simulink model "car_model"  (R2017a)
settings: Solver=ode8  StartTime=0.0  StopTime=tf  FixedStep=1e-3  RelTol=1e-3  AbsTol=1e-6
values from neighbouring files (symbols this model uses):
  sys = kinematic_model(sys)    [load_kin.m]
undefined symbols (not defined in the file or in its folder): L, MAX_DELTA, w, x0
(part 1 of 2)
settings Model: Creator=brunolnetto  LastModifiedBy=brunolnetto
settings DataIOCC: SaveState=on  StateSaveName=xoutNew  OutputSaveName=youtNew

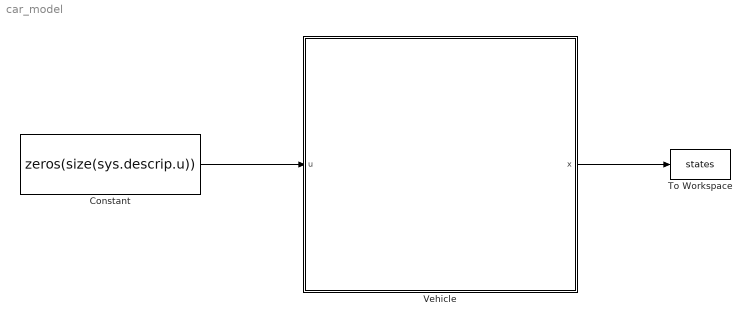
== system car_model ==
  Constant : Constant  Value=zeros(size(sys.descrip.u))
  To Workspace : ToWorkspace  VariableName=states  SaveFormat=Structure With Time  SampleTime=-1
  Vehicle : Subsystem
      mask Display: image('/home/brunolnetto/Pictures/auto_model.png');
  wires:
  Constant/1 -> Vehicle/1(u)
  Vehicle/1(x) -> To Workspace/1

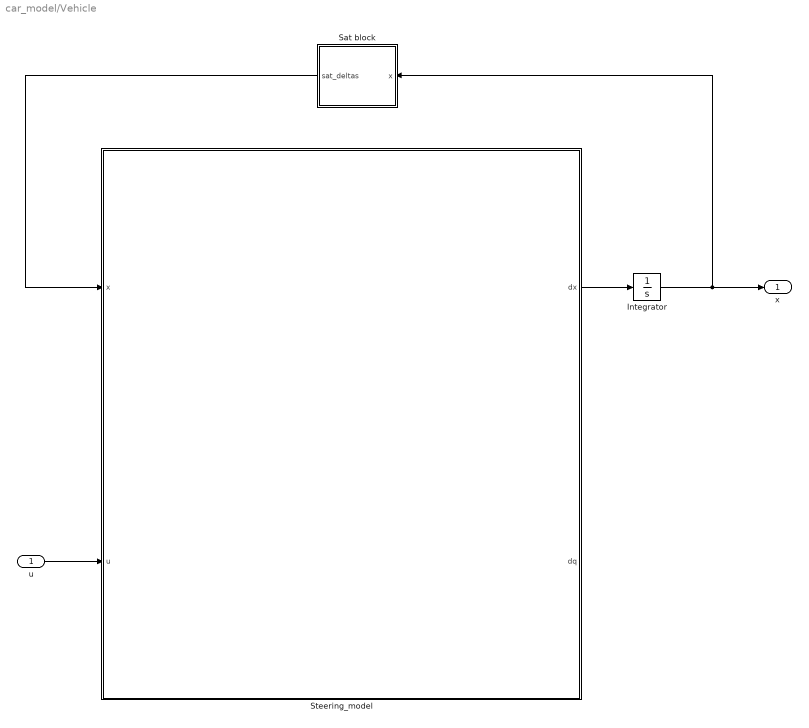
== system car_model/Vehicle ==
  u : Inport
  Integrator : Integrator  InitialCondition=x0
  Sat block : Subsystem
  Steering_model : Subsystem
      mask Display: image('/home/brunolnetto/Pictures/steer_schema.png');
  x : Outport
  wires:
  Steering_model/1(dx) -> Integrator/1
  u/1 -> Steering_model/2(u)
  Integrator/1 -> Sat block/1(x), x/1
  Sat block/1(sat_deltas) -> Steering_model/1(x)

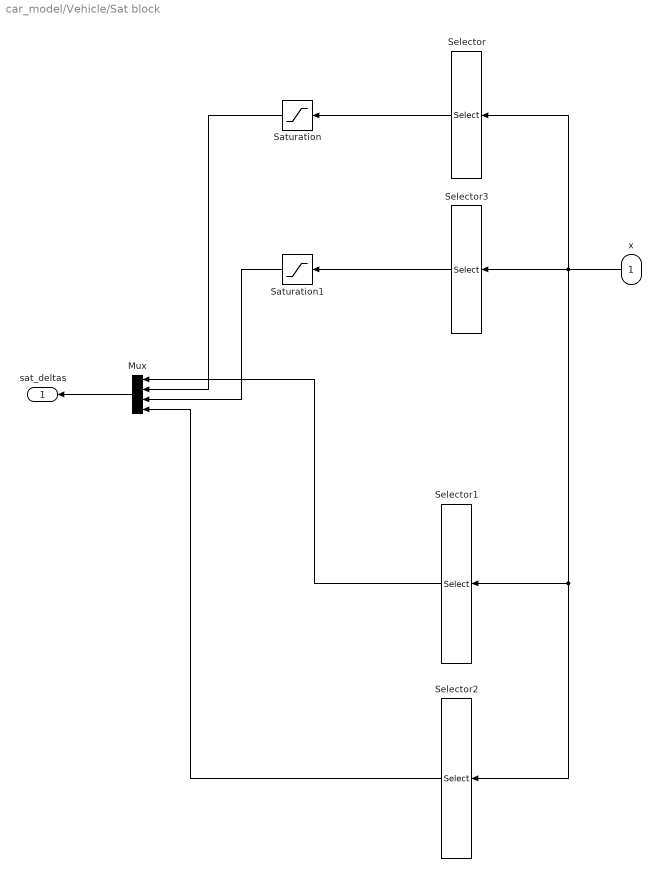
== system car_model/Vehicle/Sat block ==
  x : Inport
  Mux : Mux
  Saturation : Saturate  UpperLimit=MAX_DELTA  LowerLimit=atan(tan(-MAX_DELTA)/(1 - (w/L)*tan(-MAX_DELTA)))
  Saturation1 : Saturate  UpperLimit=atan(tan(MAX_DELTA)/(1 + (w/L)*tan(MAX_DELTA)))  LowerLimit=-MAX_DELTA
  Selector : Selector  InputPortWidth=13  IndexOptions=Index vector (dialog)  Indices=4  OutputSizes=1
  Selector1 : Selector  InputPortWidth=13  IndexOptions=Index vector (dialog)  Indices=[1 2. 3]  OutputSizes=1
  Selector2 : Selector  InputPortWidth=13  IndexOptions=Index vector (dialog)  Indices=[6. 7. 8. 9. 10. 11. 12. 13]  OutputSizes=1
  Selector3 : Selector  InputPortWidth=13  IndexOptions=Index vector (dialog)  Indices=5  OutputSizes=1
  sat_deltas : Outport
  wires:
  Selector/1 -> Saturation/1
  Mux/1 -> sat_deltas/1
  x/1 -> Selector2/1, Selector1/1, Selector3/1, Selector/1
  Selector3/1 -> Saturation1/1
  Selector2/1 -> Mux/4
  Selector1/1 -> Mux/1
  Saturation/1 -> Mux/2
  Saturation1/1 -> Mux/3

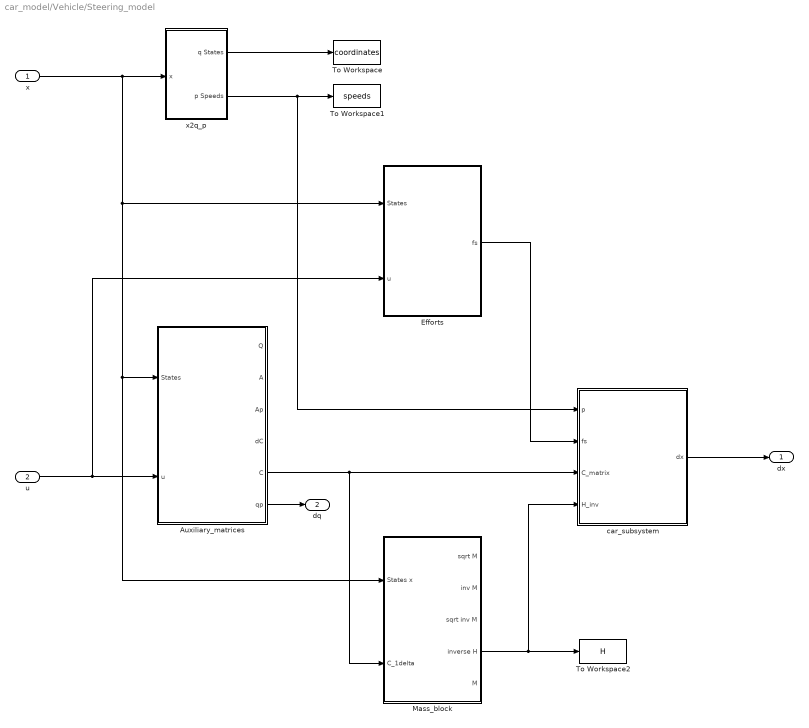
== system car_model/Vehicle/Steering_model ==
  x : Inport
  u : Inport  Port=2
  Auxiliary_matrices : Subsystem
  Efforts : Subsystem
  Mass_block : Subsystem
  To Workspace : ToWorkspace  VariableName=coordinates  SaveFormat=Structure With Time  SampleTime=-1
  To Workspace1 : ToWorkspace  VariableName=speeds  SaveFormat=Structure With Time  SampleTime=-1
  To Workspace2 : ToWorkspace  VariableName=H  SaveFormat=Structure With Time  SampleTime=-1
  car_subsystem : Subsystem
  x2q_p : Subsystem
  dx : Outport
  dq : Outport  Port=2
  wires:
  Auxiliary_matrices/5(C) -> Mass_block/2("C_1delta  "), car_subsystem/3(C_matrix)
  u/1 -> Efforts/2(u), Auxiliary_matrices/2(u)
  Mass_block/4(inverse H) -> To Workspace2/1, car_subsystem/4(H_inv)
  car_subsystem/1(dx) -> dx/1
  Efforts/1(fs) -> car_subsystem/2(fs)
  x2q_p/1(q States) -> To Workspace/1
  x2q_p/2(p Speeds) -> To Workspace1/1, car_subsystem/1(p)
  x/1 -> x2q_p/1(x), Mass_block/1(States x), Auxiliary_matrices/1(States), Efforts/1(States)
  Auxiliary_matrices/6(qp) -> dq/1

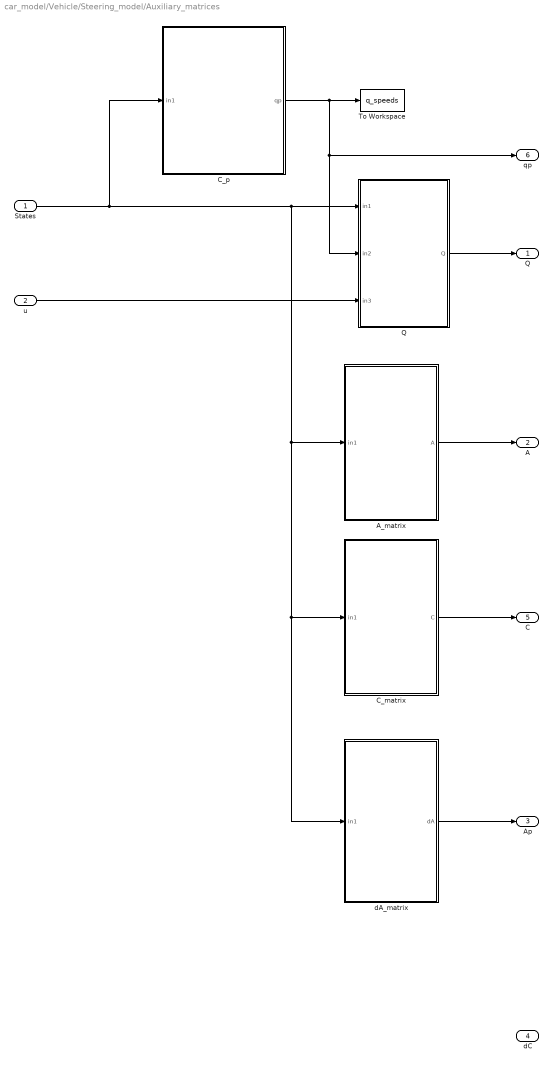
== system car_model/Vehicle/Steering_model/Auxiliary_matrices ==
  States : Inport
  u : Inport  Port=2
  A_matrix : MATLAB Function  TreatAsAtomicUnit=on
  C_matrix : MATLAB Function  TreatAsAtomicUnit=on
  C_p : MATLAB Function  TreatAsAtomicUnit=on
  Q : MATLAB Function  TreatAsAtomicUnit=on
  To Workspace : ToWorkspace  VariableName=q_speeds  SaveFormat=Structure With Time  SampleTime=-1
  dA_matrix : MATLAB Function  TreatAsAtomicUnit=on
  "Q " : Outport
  A : Outport  Port=2
  Ap : Outport  Port=3
  dC : Outport  Port=4
  C : Outport  Port=5
  qp : Outport  Port=6
  wires:
  C_matrix/1(C) -> C/1
  Q/1(Q) -> "Q "/1
  A_matrix/1(A) -> A/1
  dA_matrix/1(dA) -> Ap/1
  u/1 -> Q/3(in3)
  States/1 -> C_p/1(in1), dA_matrix/1(in1), C_matrix/1(in1), A_matrix/1(in1), Q/1(in1)
  C_p/1(qp) -> To Workspace/1, qp/1, Q/2(in2)

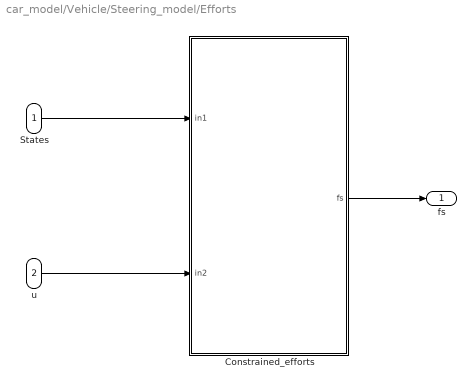
== system car_model/Vehicle/Steering_model/Efforts ==
  States : Inport
  u : Inport  Port=2
  Constrained_efforts : MATLAB Function  TreatAsAtomicUnit=on
  fs : Outport
  wires:
  States/1 -> Constrained_efforts/1(in1)
  u/1 -> Constrained_efforts/2(in2)
  Constrained_efforts/1(fs) -> fs/1

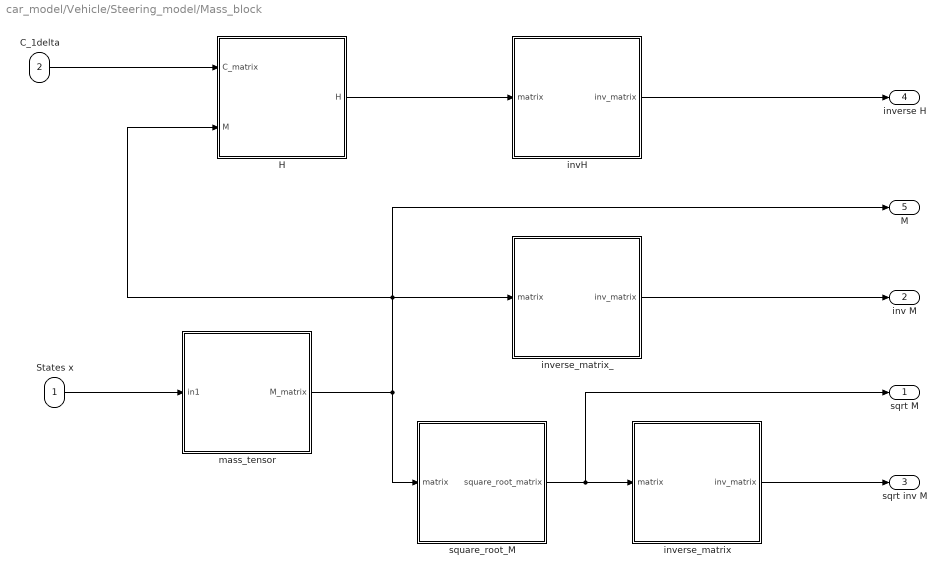
== system car_model/Vehicle/Steering_model/Mass_block ==
  States x : Inport
  "C_1delta  " : Inport  Port=2
  H : MATLAB Function  TreatAsAtomicUnit=on
  invH : MATLAB Function  TreatAsAtomicUnit=on
  inverse_matrix : MATLAB Function  TreatAsAtomicUnit=on
  inverse_matrix_ : MATLAB Function  TreatAsAtomicUnit=on
  mass_tensor : MATLAB Function  TreatAsAtomicUnit=on
  square_root_M : MATLAB Function  TreatAsAtomicUnit=on
  sqrt M : Outport
  inv M : Outport  Port=2
  sqrt inv M : Outport  Port=3
  inverse H : Outport  Port=4
  M : Outport  Port=5
  wires:
  States x/1 -> mass_tensor/1(in1)
  "C_1delta  "/1 -> H/1(C_matrix)
  inverse_matrix_/1(inv_matrix) -> inv M/1
  H/1(H) -> invH/1(matrix)
  invH/1(inv_matrix) -> inverse H/1
  inverse_matrix/1(inv_matrix) -> sqrt inv M/1
  mass_tensor/1(M_matrix) -> M/1, inverse_matrix_/1(matrix), H/2(M), square_root_M/1(matrix)
  square_root_M/1(square_root_matrix) -> sqrt M/1, inverse_matrix/1(matrix)

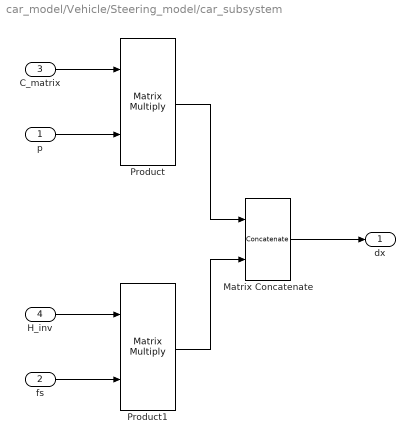
== system car_model/Vehicle/Steering_model/car_subsystem ==
  p : Inport
  fs : Inport  Port=2
  C_matrix : Inport  Port=3
  H_inv : Inport  Port=4
  Matrix Concatenate : Concatenate  ConcatenateDimension=2
  Product : Product  Multiplication=Matrix(*)
  Product1 : Product  Multiplication=Matrix(*)
  dx : Outport
  wires:
  Product/1 -> Matrix Concatenate/1
  p/1 -> Product/2
  C_matrix/1 -> Product/1
  Product1/1 -> Matrix Concatenate/2
  H_inv/1 -> Product1/1
  fs/1 -> Product1/2
  Matrix Concatenate/1 -> dx/1

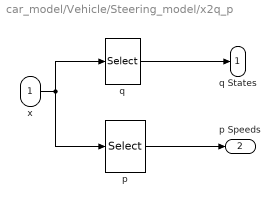
== system car_model/Vehicle/Steering_model/x2q_p ==
  x : Inport
  p : Selector  InputPortWidth=13  IndexOptions=Index vector (dialog)  Indices=[10 11 12 13]  OutputSizes=1
  q : Selector  InputPortWidth=13  IndexOptions=Index vector (dialog)  Indices=[1 2 3 4 5 6 7 8 9]  OutputSizes=1
  q States : Outport
  p Speeds : Outport  Port=2
  wires:
  x/1 -> p/1, q/1
  q/1 -> q States/1
  p/1 -> p Speeds/1

== matlab function car_model/Vehicle/Steering_model/Auxiliary_matrices/A_matrix ==
  data: in1 input; A output
function A = ConstraintMatrix(in1)

%    This function was generated by the Symbolic Math Toolbox version 7.2.

%    11-Nov-2020 11:00:00



delta_o = in1(5,:);

theta = in1(3,:);

t2 = tan(theta);

t3 = tan(delta_o);

t4 = t2.*(3.0./2.0);

t5 = t4+9.0./2.0;

t6 = 1.0./t5;

t7 = t2.^2;

t8 = 1.0./t5.^2;

t9 = t7.*t8.*(8.1e1./4.0);

t10 = t9+1.0;

t11 = t2.*t6.*(2.7e1./4.0);

t12 = t2.*t6.*(9.0./2.0);

t13 = atan(t12);

t14 = t13+theta;

t15 = 1.0./sqrt(t10);

t16 = sin(t14);

t17 = cos(t14);

A = reshape([0.0,0.0,0.0,t17,-t16,0.0,0.0,0.0,t16,t17,0.0,0.0,0.0,t15.*(-9.0./2.0)+t2.*t6.*t15.*(2.7e1./8.0),t15.*(3.0./4.0)+t2.*t6.*t15.*(8.1e1./4.0),t10.*(t3.*(3.0./2.0)-9.0./2.0).*(-2.0./9.0),0.0,0.0,0.0,0.0,(t3.^2+1.0).*(t11+9.0./2.0).*(-2.0./9.0),0.0,0.0,0.0,0.0,0.0,0.0,sqrt(t10),-3.442462000000001e-1,0.0,0.0,0.0,(t11-9.0)./(cos(delta_o).*(t11+9.0)),0.0,0.0,0.0,t2.*t6.*(-3.0./2.0)-1.0,0.0,0.0,0.0,0.0,1.0,0.0,0.0,0.0],[5,9]);

end

== matlab function car_model/Vehicle/Steering_model/Mass_block/mass_tensor ==
  data: in1 input; M_matrix output
function M_matrix = Mass_matrix(in1)

%    This function was generated by the Symbolic Math Toolbox version 7.2.

%    11-Nov-2020 11:00:06



delta_o = in1(5,:);

phi_i = in1(6,:);

phi_l = in1(9,:);

phi_o = in1(7,:);

phi_r = in1(8,:);

theta = in1(3,:);

t2 = cos(theta);

t3 = sin(theta);

t4 = cos(phi_i);

t5 = t4.^2;

t6 = cos(phi_l);

t7 = t6.^2;

t8 = cos(phi_o);

t9 = t8.^2;

t10 = cos(phi_r);

t11 = t10.^2;

t12 = t2.^2;

t13 = sin(phi_l);

t14 = t13.^2;

t15 = sin(phi_r);

t16 = t15.^2;

t17 = t3.^2;

t18 = cos(delta_o);

t19 = sin(phi_o);

t20 = t19.^2;

t21 = t18.^2;

t22 = sin(delta_o);

t23 = t22.^2;

t24 = t20.^2;

t25 = sin(phi_i);

t26 = t25.^2;

t27 = tan(theta);

t28 = t27.^2;

t29 = t27.*(3.0./2.0);

t30 = t29+9.0./2.0;

t31 = 1.0./t30.^2;

t32 = t28.*t31.*(8.1e1./4.0);

t33 = t32+1.0;

t34 = 1.0./t33;

t35 = t26.^2;

t36 = 1.0./sqrt(t33);

t37 = 1.0./t30;

t38 = phi_i.*4.0;

t39 = cos(t38);

t40 = t5.^2;

t41 = t40.*4.147690617505401e-1;

t42 = t12.*t34.*t35.*4.147690617505401e-1;

t43 = t17.*t26.*t34.*2.073845308752701e-1;

t44 = t5.*t12.*t26.*t34.*2.073845308752701e-1;

t45 = t12.*t26.*t28.*t31.*t34.*4.199536750224219;

t46 = t17.*t28.*t31.*t34.*t35.*8.399073500448438;

t47 = t3.*t5.*t26.*t27.*t36.*t37.*1.866460777877431;

t48 = t2.*t3.*t26.*t27.*t34.*t37.*1.866460777877431;

t49 = t5.*t17.*t26.*t28.*t31.*t34.*4.199536750224219;

t50 = phi_o.*4.0;

t51 = cos(t50);

t52 = t9.^2;

t53 = t52.*4.147690617505401e-1;

t54 = t12.*t21.*t24.*4.147690617505401e-1;

t55 = t17.*t20.*t21.*2.073845308752701e-1;

t56 = t12.*t20.*t23.*2.073845308752701e-1;

t57 = t17.*t23.*t24.*4.147690617505401e-1;

t58 = t9.*t12.*t20.*t21.*2.073845308752701e-1;

t59 = t9.*t17.*t20.*t23.*2.073845308752701e-1;

t60 = t3.*t9.*t20.*t22.*4.147690617505401e-1;

t61 = t2.*t3.*t18.*t20.*t22.*4.147690617505401e-1;

t62 = phi_i.*3.0;

t63 = sin(t62);

t64 = theta.*2.0;

t65 = t27.*t37.*(9.0./2.0);

t66 = atan(t65);

t67 = t66.*2.0;

t68 = cos(t64);

t69 = sin(t67);

t70 = sin(t64);

t71 = cos(t67);

t72 = delta_o.*2.0;

t73 = phi_o.*3.0;

t74 = sin(t73);

t75 = cos(t72);

t76 = sin(t72);

t78 = t39.*2.592306635940876e-2;

t79 = t2.*t5.*t26.*t36.*4.147690617505401e-1;

t80 = t2.*t3.*t27.*t34.*t35.*t37.*3.732921555754861;

t81 = t2.*t3.*t5.*t26.*t27.*t34.*t37.*1.866460777877431;

t77 = t41+t42+t43+t44+t45+t46+t47+t48+t49-t78-t79-t80-t81+2.592306635940876e-2;

t82 = t63.*t68.*t69.*2.592306635940876e-2;

t83 = t63.*t70.*t71.*2.592306635940876e-2;

t84 = t3.*t25.*t36.*5.184613271881752e-2;

t85 = t3.*t36.*t63.*5.184613271881752e-2;

t86 = t2.*t25.*t27.*t36.*t37.*2.333075972346788e-1;

t87 = t2.*t27.*t36.*t37.*t63.*2.333075972346788e-1;

t101 = t25.*t68.*t69.*7.776919907822627e-2;

t102 = t25.*t70.*t71.*7.776919907822627e-2;

t88 = t82+t83+t84+t85+t86+t87-t101-t102;

t90 = t51.*2.592306635940876e-2;

t91 = t2.*t9.*t18.*t20.*4.147690617505401e-1;

t92 = t2.*t3.*t18.*t22.*t24.*8.295381235010802e-1;

t93 = t2.*t3.*t9.*t18.*t20.*t22.*4.147690617505401e-1;

t89 = t53+t54+t55+t56+t57+t58+t59+t60+t61-t90-t91-t92-t93+2.592306635940876e-2;

t94 = t70.*t74.*t75.*2.592306635940876e-2;

t95 = t68.*t74.*t76.*2.592306635940876e-2;

t96 = t3.*t18.*t74.*5.184613271881752e-2;

t97 = t2.*t22.*t74.*5.184613271881752e-2;

t98 = t3.*t18.*t19.*5.184613271881752e-2;

t99 = t2.*t19.*t22.*5.184613271881752e-2;

t103 = t19.*t70.*t75.*7.776919907822627e-2;

t104 = t19.*t68.*t76.*7.776919907822627e-2;

t100 = t94+t95+t96+t97+t98+t99-t103-t104;

t105 = t2.*t3.*t15.*2.073845308752701e-1;

t106 = t3.*t11.*t15.*2.073845308752701e-1;

t107 = t105+t106-t2.*t3.*t11.*t15.*2.073845308752701e-1-t2.*t3.*t15.*t16.*4.147690617505401e-1;

t108 = t2.*t3.*t13.*2.073845308752701e-1;

t109 = t3.*t7.*t13.*2.073845308752701e-1;

t110 = t108+t109-t2.*t3.*t7.*t13.*2.073845308752701e-1-t2.*t3.*t13.*t14.*4.147690617505401e-1;

t111 = t12.*2.073845308752701e-1;

M_matrix = reshape([1.885e3,0.0,t2.*(-4.24125e3),0.0,0.0,0.0,0.0,0.0,0.0,0.0,1.885e3,t3.*(-4.24125e3),0.0,0.0,0.0,0.0,0.0,0.0,t2.*(-4.24125e3),t3.*(-4.24125e3),t12.*9.7003125e3+t17.*9.7003125e3-t39.*2.592306635940876e-2+t41+t42+t43+t44+t45+t46+t47+t48+t49-t51.*2.592306635940876e-2+t53+t54+t55+t56+t57+t58+t59+t60+t61-cos(phi_l.*4.0).*2.592306635940876e-2-cos(phi_r.*4.0).*2.592306635940876e-2+t14.*t17.*2.073845308752701e-1+t16.*t17.*2.073845308752701e-1+t12.*t14.^2.*4.147690617505401e-1+t12.*t16.^2.*4.147690617505401e-1+t7.^2.*4.147690617505401e-1+t11.^2.*4.147690617505401e-1+t2.*t7.*(t7-1.0).*4.147690617505401e-1+t2.*t11.*(t11-1.0).*4.147690617505401e-1+t7.*t12.*t14.*2.073845308752701e-1+t11.*t12.*t16.*2.073845308752701e-1-t2.*t9.*t18.*t20.*4.147690617505401e-1-t2.*t5.*t26.*t36.*4.147690617505401e-1-t2.*t3.*t18.*t22.*t24.*8.295381235010802e-1-t2.*t3.*t9.*t18.*t20.*t22.*4.147690617505401e-1-t2.*t3.*t27.*t34.*t35.*t37.*3.732921555754861-t2.*t3.*t5.*t26.*t27.*t34.*t37.*1.866460777877431+3.481978692265438e3,t77,t89,t88,t100,t107,t110,0.0,0.0,t77,t77,0.0,t88,0.0,0.0,0.0,0.0,0.0,t89,0.0,t89,0.0,t100,0.0,0.0,0.0,0.0,t88,t88,0.0,t5.*(-1.03692265437635e-1)-t68.*t71.*1.03692265437635e-1+t69.*t70.*1.03692265437635e-1+t5.*t68.*t71.*1.03692265437635e-1-t5.*t69.*t70.*1.03692265437635e-1+3.110767963129051e-1,0.0,0.0,0.0,0.0,0.0,t100,0.0,t100,0.0,t9.*(-1.03692265437635e-1)-t68.*t75.*1.03692265437635e-1+t70.*t76.*1.03692265437635e-1+t9.*t68.*t75.*1.03692265437635e-1-t9.*t70.*t76.*1.03692265437635e-1+3.110767963129051e-1,0.0,0.0,0.0,0.0,t107,0.0,0.0,0.0,0.0,t111+t11.*t17.*2.073845308752701e-1+t16.*t17.*4.147690617505401e-1,0.0,0.0,0.0,t110,0.0,0.0,0.0,0.0,0.0,t111+t7.*t17.*2.073845308752701e-1+t14.*t17.*4.147690617505401e-1],[9,9]);

end

== matlab function car_model/Vehicle/Steering_model/Auxiliary_matrices/C_matrix ==
  data: in1 input; C output
function C = KinematicMatrix(in1)

%    This function was generated by the Symbolic Math Toolbox version 7.2.

%    11-Nov-2020 11:00:01



delta_o = in1(5,:);

theta = in1(3,:);

t2 = tan(theta);

t3 = t2.^2;

t4 = t2.*(3.0./2.0);

t5 = t4+9.0./2.0;

t6 = 1.0./t5.^2;

t7 = t3.*t6.*(8.1e1./4.0);

t8 = t7+1.0;

t9 = 1.0./sqrt(t8);

t10 = 1.0./t5;

t11 = t2.*t10.*(9.0./2.0);

t12 = atan(t11);

t13 = t12.*2.0;

t14 = t13+theta;

t15 = cos(theta);

t16 = t15.*(9.0./2.0);

t17 = sin(theta);

t18 = t17.*(3.0./4.0);

t19 = cos(delta_o);

t20 = 1.0./t19;

t21 = t9.*9.0;

t22 = t2.*t9.*t10.*(2.7e1./4.0);

t23 = t21+t22;

t24 = 1.0./t23;

t25 = cos(t14);

t26 = sin(t14);

t27 = t17.*(9.0./2.0);

t28 = delta_o.*2.0;

C = reshape([t16+t18,t15.*(-3.0./4.0)+t27,1.0,0.0,0.0,0.0,0.0,0.0,0.0,0.0,0.0,0.0,(cos(t13).*(9.0./2.0)+sin(t13).*(3.0./2.0)+9.0./2.0)./(cos(t28).*(9.0./2.0)-sin(t28).*(3.0./2.0)+9.0./2.0),1.0,0.0,0.0,0.0,0.0,t9.*t20.*t24.*(t16+t18+t25.*(9.0./2.0)-t26.*(3.0./4.0)).*3.442462000000001e-1,t9.*t20.*t24.*(t15.*(-3.0./4.0)+t25.*(3.0./4.0)+t26.*(9.0./2.0)+t27).*3.442462000000001e-1,0.0,0.0,0.0,t9.*t20.*t24.*(t21-t22),1.0,0.0,0.0,0.0,0.0,0.0,0.0,0.0,0.0,0.0,(9.0./2.0)./(t2.*t10.*(2.7e1./4.0)+9.0./2.0),1.0],[9,4]);

end

== matlab function car_model/Vehicle/Steering_model/Auxiliary_matrices/Q ==
  data: in1 input; in2 input; in3 input; Q output
function Q = EffortVector(in1,in2,in3)

%    This function was generated by the Symbolic Math Toolbox version 7.2.

%    11-Nov-2020 10:59:58



delta_o = in1(5,:);

deltap_i = in2(4,:);

deltap_o = in2(5,:);

f_phi_i = in3(1,:);

f_phi_l = in3(4,:);

f_phi_o = in3(2,:);

f_phi_r = in3(3,:);

phi_i = in1(6,:);

phi_l = in1(9,:);

phi_o = in1(7,:);

phi_r = in1(8,:);

phip_i = in2(6,:);

phip_l = in2(9,:);

phip_o = in2(7,:);

phip_r = in2(8,:);

thetap = in2(3,:);

theta = in1(3,:);

t2 = thetap.^2;

t3 = sin(theta);

t4 = tan(theta);

t5 = t4.*(3.0./2.0);

t6 = t5+9.0./2.0;

t7 = 1.0./t6;

t8 = t4.*t7.*(9.0./2.0);

t9 = atan(t8);

t10 = t9+theta;

t11 = sin(t10);

t12 = phip_l.^2;

t13 = theta.*2.0;

t14 = phip_r.^2;

t15 = phip_o.^2;

t16 = delta_o.*2.0;

t17 = deltap_o.^2;

t18 = phi_o.*2.0;

t19 = t13+t16+t18;

t20 = sin(t19);

t21 = t13+t16-t18;

t22 = sin(t21);

t23 = phi_o.*4.0;

t24 = t13+t16+t23;

t25 = sin(t24);

t26 = sin(t13);

t27 = phip_i.^2;

t28 = t13+t16;

t29 = sin(t28);

t30 = phi_l.*2.0;

t31 = phi_l.*3.0;

t32 = phi_r.*2.0;

t33 = phi_r.*3.0;

t34 = -t13+t30;

t35 = sin(t34);

t36 = t13+t30;

t37 = sin(t36);

t38 = phi_l.*4.0;

t39 = -t13+t32;

t40 = sin(t39);

t41 = t13+t32;

t42 = sin(t41);

t43 = phi_r.*4.0;

t44 = deltap_i.^2;

t45 = t9.*2.0;

t46 = phi_o.*3.0;

t47 = delta_o-t23+theta;

t48 = sin(t47);

t49 = delta_o+t23+theta;

t50 = sin(t49);

t51 = phi_i.*2.0;

t52 = t13+t45+t51;

t53 = sin(t52);

t54 = t13+t45-t51;

t55 = sin(t54);

t56 = phi_i.*4.0;

t57 = t13+t45+t56;

t58 = sin(t57);

t59 = delta_o+theta;

t60 = sin(t59);

t61 = t13+t45;

t62 = sin(t61);

t63 = phi_i.*3.0;

t64 = t9-t56+theta;

t65 = sin(t64);

t66 = t9+t56+theta;

t67 = sin(t66);

t68 = t38+theta;

t69 = sin(t68);

t70 = t43+theta;

t71 = sin(t70);

t72 = t13+t16-t23;

t73 = sin(t72);

t74 = sin(t51);

t75 = sin(t56);

t76 = sin(t18);

t77 = sin(t23);

t78 = t38-theta;

t79 = sin(t78);

t80 = -t13+t38;

t81 = sin(t80);

t82 = t13+t38;

t83 = sin(t82);

t84 = t43-theta;

t85 = sin(t84);

t86 = -t13+t43;

t87 = sin(t86);

t88 = t13+t43;

t89 = sin(t88);

t90 = t13+t45-t56;

t91 = sin(t90);

t92 = phi_i+t13+t45;

t93 = sin(t92);

t94 = t27.*t93.*3.888459953911314e-2;

t95 = phi_i+t9+theta;

t96 = sin(t95);

t97 = t44.*t58.*6.480766589852189e-3;

t98 = -phi_i+t13+t45;

t99 = sin(t98);

t100 = t27.*t99.*3.888459953911314e-2;

t101 = t13+t45+t63;

t102 = sin(t101);

t103 = t2.*t91.*6.480766589852189e-3;

t104 = t2.*t58.*6.480766589852189e-3;

t105 = t44.*t62.*3.888459953911314e-2;

t106 = t27.*t62.*5.184613271881752e-2;

t107 = t2.*t62.*3.888459953911314e-2;

t108 = t44.*t65.*1.296153317970438e-2;

t109 = t44.*t67.*1.296153317970438e-2;

t110 = -phi_i+t9+theta;

t111 = sin(t110);

t112 = t9-t63+theta;

t113 = sin(t112);

t114 = t9+t63+theta;

t115 = sin(t114);

t116 = t2.*t65.*1.296153317970438e-2;

t117 = t2.*t67.*1.296153317970438e-2;

t118 = deltap_i.*t65.*thetap.*2.592306635940876e-2;

t119 = deltap_i.*t67.*thetap.*2.592306635940876e-2;

t120 = phip_i.*t67.*thetap.*1.03692265437635e-1;

t121 = deltap_i.*phip_i.*t74.*1.03692265437635e-1;

t122 = deltap_i.*phip_i.*t75.*1.555383981564525e-1;

t123 = phip_i.*t74.*thetap.*1.03692265437635e-1;

t124 = phip_i.*t75.*thetap.*1.555383981564525e-1;

t125 = deltap_i.*phip_i.*t55.*5.184613271881752e-2;

t126 = deltap_i.*phip_i.*t58.*2.592306635940876e-2;

t127 = deltap_i.*t91.*thetap.*1.296153317970438e-2;

t128 = deltap_i.*t58.*thetap.*1.296153317970438e-2;

t129 = phip_i.*t55.*thetap.*5.184613271881752e-2;

t130 = phip_i.*t58.*thetap.*2.592306635940876e-2;

t131 = deltap_i.*t62.*thetap.*7.776919907822627e-2;

t132 = deltap_i.*phip_i.*t67.*1.03692265437635e-1;

t133 = phi_o+t13+t16;

t134 = sin(t133);

t135 = t15.*t134.*3.888459953911314e-2;

t136 = delta_o+phi_o+theta;

t137 = sin(t136);

t138 = t17.*t25.*6.480766589852189e-3;

t139 = -phi_o+t13+t16;

t140 = sin(t139);

t141 = t15.*t140.*3.888459953911314e-2;

t142 = t13+t16+t46;

t143 = sin(t142);

t144 = t2.*t73.*6.480766589852189e-3;

t145 = t2.*t25.*6.480766589852189e-3;

t146 = t17.*t29.*3.888459953911314e-2;

t147 = t15.*t29.*5.184613271881752e-2;

t148 = t2.*t29.*3.888459953911314e-2;

t149 = t17.*t48.*1.296153317970438e-2;

t150 = t17.*t50.*1.296153317970438e-2;

t151 = delta_o-phi_o+theta;

t152 = sin(t151);

t153 = delta_o-t46+theta;

t154 = sin(t153);

t155 = delta_o+t46+theta;

t156 = sin(t155);

t157 = t2.*t48.*1.296153317970438e-2;

t158 = t2.*t50.*1.296153317970438e-2;

t159 = deltap_o.*phip_o.*t22.*5.184613271881752e-2;

t160 = deltap_o.*phip_o.*t25.*2.592306635940876e-2;

t161 = deltap_o.*t73.*thetap.*1.296153317970438e-2;

t162 = deltap_o.*t25.*thetap.*1.296153317970438e-2;

t163 = deltap_o.*phip_o.*t76.*1.03692265437635e-1;

t164 = deltap_o.*phip_o.*t77.*1.555383981564525e-1;

t165 = phip_o.*t22.*thetap.*5.184613271881752e-2;

t166 = phip_o.*t25.*thetap.*2.592306635940876e-2;

t167 = phip_o.*t76.*thetap.*1.03692265437635e-1;

t168 = phip_o.*t77.*thetap.*1.555383981564525e-1;

t169 = deltap_o.*t29.*thetap.*7.776919907822627e-2;

t170 = deltap_o.*phip_o.*t50.*1.03692265437635e-1;

t171 = deltap_o.*t48.*thetap.*2.592306635940876e-2;

t172 = deltap_o.*t50.*thetap.*2.592306635940876e-2;

t173 = phip_o.*t50.*thetap.*1.03692265437635e-1;

t174 = cos(t13);

t175 = cos(t45);

t176 = sin(t63);

t177 = sin(t45);

t178 = cos(theta);

t179 = sin(phi_i);

t180 = t4.^2;

t181 = 1.0./t6.^2;

t182 = t180.*t181.*(8.1e1./4.0);

t183 = t182+1.0;

t184 = 1.0./sqrt(t183);

t185 = cos(t51);

t186 = cos(delta_o);

t187 = sin(t46);

t188 = sin(delta_o);

t189 = cos(t16);

t190 = sin(phi_o);

t191 = sin(t16);

t192 = cos(t18);

t193 = sin(phi_r);

t194 = t193.^2;

t195 = cos(phi_r);

t196 = t195.^2;

t197 = t178.^2;

t198 = t3.^2;

t199 = sin(phi_l);

t200 = t199.^2;

t201 = cos(phi_l);

t202 = t201.^2;

Q = [t2.*t3.*(-4.24125e3);t2.*t178.*4.24125e3;t94+t97+t100+t103+t104+t105+t106+t107+t108+t109+t116+t117+t118+t119+t120+t121+t122+t123+t124+t125+t126+t127+t128+t129+t130+t131+t132+t135+t138+t141+t144+t145+t146+t147+t148+t149+t150+t157+t158+t159+t160+t161+t162+t163+t164+t165+t166+t167+t168+t169+t170+t171+t172+t173-t2.*t3.*5.184613271881752e-2-t2.*t11.*2.592306635940876e-2-t2.*t20.*2.592306635940876e-2-t2.*t22.*2.592306635940876e-2+t2.*t26.*7.776919907822627e-2-t15.*t20.*2.592306635940876e-2+t2.*t35.*2.592306635940876e-2-t15.*t22.*2.592306635940876e-2-t17.*t20.*2.592306635940876e-2+t12.*t26.*5.184613271881752e-2-t2.*t37.*2.592306635940876e-2+t14.*t26.*5.184613271881752e-2+t2.*t40.*2.592306635940876e-2-t2.*t42.*2.592306635940876e-2+t12.*t35.*2.592306635940876e-2-t12.*t37.*2.592306635940876e-2+t14.*t40.*2.592306635940876e-2-t2.*t53.*2.592306635940876e-2-t11.*t44.*2.592306635940876e-2-t14.*t42.*2.592306635940876e-2-t2.*t55.*2.592306635940876e-2-t2.*t60.*2.592306635940876e-2+t2.*t69.*1.296153317970438e-2+t2.*t71.*1.296153317970438e-2-t17.*t60.*2.592306635940876e-2-t27.*t53.*2.592306635940876e-2-t2.*t79.*1.296153317970438e-2-t27.*t55.*2.592306635940876e-2-t2.*t81.*6.480766589852189e-3+t2.*t83.*6.480766589852189e-3-t2.*t85.*1.296153317970438e-2-t2.*t87.*6.480766589852189e-3+t2.*t89.*6.480766589852189e-3-t44.*t53.*2.592306635940876e-2-t27.*t96.*2.592306635940876e-2-t27.*t102.*3.888459953911314e-2-t27.*t111.*2.592306635940876e-2-t27.*t113.*7.776919907822627e-2-t27.*t115.*7.776919907822627e-2-t15.*t137.*2.592306635940876e-2-t15.*t143.*3.888459953911314e-2-t15.*t152.*2.592306635940876e-2-t15.*t154.*7.776919907822627e-2-t15.*t156.*7.776919907822627e-2-t15.*sin(phi_o.*-3.0+t13+t16).*3.888459953911314e-2-t17.*sin(phi_o.*-2.0+t13+t16).*2.592306635940876e-2+t17.*sin(phi_o.*-4.0+t13+t16).*6.480766589852189e-3-t27.*sin(phi_i.*-3.0+t13+t45).*3.888459953911314e-2-t44.*sin(phi_i.*-2.0+t13+t45).*2.592306635940876e-2+t44.*sin(phi_i.*-4.0+t13+t45).*6.480766589852189e-3+t12.*sin(phi_l+t13).*3.888459953911314e-2+t14.*sin(phi_r+t13).*3.888459953911314e-2-t12.*sin(phi_l+theta).*2.592306635940876e-2-t14.*sin(phi_r+theta).*2.592306635940876e-2-t12.*sin(t13+t31).*3.888459953911314e-2-t14.*sin(t13+t33).*3.888459953911314e-2-t12.*sin(t31+theta).*7.776919907822627e-2-t14.*sin(t33+theta).*7.776919907822627e-2-t12.*sin(phi_l-t13).*3.888459953911314e-2-t14.*sin(phi_r-t13).*3.888459953911314e-2+t12.*sin(phi_l-theta).*2.592306635940876e-2+t14.*sin(phi_r-theta).*2.592306635940876e-2+t12.*sin(-t13+t31).*3.888459953911314e-2+t14.*sin(-t13+t33).*3.888459953911314e-2+t12.*sin(t31-theta).*7.776919907822627e-2+t14.*sin(t33-theta).*7.776919907822627e-2+phip_l.*thetap.*sin(t30).*1.03692265437635e-1+phip_l.*thetap.*sin(t38).*1.555383981564525e-1+phip_r.*thetap.*sin(t32).*1.03692265437635e-1+phip_r.*thetap.*sin(t43).*1.555383981564525e-1-deltap_o.*phip_o.*t20.*5.184613271881752e-2-deltap_i.*phip_i.*t53.*5.184613271881752e-2-deltap_o.*phip_o.*t48.*1.03692265437635e-1-deltap_i.*phip_i.*t65.*1.03692265437635e-1-deltap_o.*phip_o.*t73.*2.592306635940876e-2-deltap_i.*phip_i.*t91.*2.592306635940876e-2-deltap_i.*t11.*thetap.*5.184613271881752e-2-deltap_o.*t20.*thetap.*5.184613271881752e-2-deltap_o.*t22.*thetap.*5.184613271881752e-2-deltap_i.*t53.*thetap.*5.184613271881752e-2-deltap_i.*t55.*thetap.*5.184613271881752e-2-deltap_o.*t60.*thetap.*5.184613271881752e-2-phip_o.*t20.*thetap.*5.184613271881752e-2-phip_l.*t35.*thetap.*5.184613271881752e-2-phip_l.*t37.*thetap.*5.184613271881752e-2-phip_r.*t40.*thetap.*5.184613271881752e-2-phip_r.*t42.*thetap.*5.184613271881752e-2-phip_i.*t53.*thetap.*5.184613271881752e-2-phip_o.*t48.*thetap.*1.03692265437635e-1-phip_i.*t65.*thetap.*1.03692265437635e-1+phip_l.*t69.*thetap.*1.03692265437635e-1-phip_o.*t73.*thetap.*2.592306635940876e-2+phip_r.*t71.*thetap.*1.03692265437635e-1+phip_l.*t79.*thetap.*1.03692265437635e-1+phip_l.*t81.*thetap.*2.592306635940876e-2+phip_l.*t83.*thetap.*2.592306635940876e-2-phip_i.*t91.*thetap.*2.592306635940876e-2+phip_r.*t85.*thetap.*1.03692265437635e-1+phip_r.*t87.*thetap.*2.592306635940876e-2+phip_r.*t89.*thetap.*2.592306635940876e-2;t94+t97+t100+t103+t104+t105+t106+t107+t108+t109+t116+t117+t118+t119+t120+t121+t122+t123+t124+t125+t126+t127+t128+t129+t130+t131+t132-t2.*t11.*2.592306635940876e-2-t2.*t53.*2.592306635940876e-2-t11.*t44.*2.592306635940876e-2-t2.*t55.*2.592306635940876e-2-t27.*t53.*2.592306635940876e-2-t27.*t55.*2.592306635940876e-2-t44.*t53.*2.592306635940876e-2-t44.*t55.*2.592306635940876e-2-t27.*t96.*2.592306635940876e-2-t27.*t102.*3.888459953911314e-2+t44.*t91.*6.480766589852189e-3-t27.*t111.*2.592306635940876e-2-t27.*t113.*7.776919907822627e-2-t27.*t115.*7.776919907822627e-2-t27.*sin(t13+t45-t63).*3.888459953911314e-2-deltap_i.*phip_i.*t53.*5.184613271881752e-2-deltap_i.*phip_i.*t65.*1.03692265437635e-1-deltap_i.*phip_i.*t91.*2.592306635940876e-2-deltap_i.*t11.*thetap.*5.184613271881752e-2-deltap_i.*t53.*thetap.*5.184613271881752e-2-deltap_i.*t55.*thetap.*5.184613271881752e-2-phip_i.*t53.*thetap.*5.184613271881752e-2-phip_i.*t65.*thetap.*1.03692265437635e-1-phip_i.*t91.*thetap.*2.592306635940876e-2;t135+t138+t141+t144+t145+t146+t147+t148+t149+t150+t157+t158+t159+t160+t161+t162+t163+t164+t165+t166+t167+t168+t169+t170+t171+t172+t173-t2.*t20.*2.592306635940876e-2-t2.*t22.*2.592306635940876e-2-t15.*t20.*2.592306635940876e-2-t15.*t22.*2.592306635940876e-2-t17.*t20.*2.592306635940876e-2-t17.*t22.*2.592306635940876e-2-t2.*t60.*2.592306635940876e-2-t17.*t60.*2.592306635940876e-2+t17.*t73.*6.480766589852189e-3-t15.*t137.*2.592306635940876e-2-t15.*t143.*3.888459953911314e-2-t15.*t152.*2.592306635940876e-2-t15.*t154.*7.776919907822627e-2-t15.*t156.*7.776919907822627e-2-t15.*sin(t13+t16-t46).*3.888459953911314e-2-deltap_o.*phip_o.*t20.*5.184613271881752e-2-deltap_o.*phip_o.*t48.*1.03692265437635e-1-deltap_o.*phip_o.*t73.*2.592306635940876e-2-deltap_o.*t20.*thetap.*5.184613271881752e-2-deltap_o.*t22.*thetap.*5.184613271881752e-2-deltap_o.*t60.*thetap.*5.184613271881752e-2-phip_o.*t20.*thetap.*5.184613271881752e-2-phip_o.*t48.*thetap.*1.03692265437635e-1-phip_o.*t73.*thetap.*2.592306635940876e-2;f_phi_i-t2.*t74.*5.184613271881752e-2-t2.*t75.*7.776919907822627e-2-t27.*t74.*5.184613271881752e-2-t44.*t74.*5.184613271881752e-2-t44.*t75.*7.776919907822627e-2-deltap_i.*t74.*thetap.*1.03692265437635e-1-deltap_i.*t75.*thetap.*1.555383981564525e-1-deltap_i.*phip_i.*t26.*t175.*1.03692265437635e-1-deltap_i.*phip_i.*t174.*t177.*1.03692265437635e-1-phip_i.*t26.*t175.*thetap.*1.03692265437635e-1-phip_i.*t174.*t177.*thetap.*1.03692265437635e-1-t2.*t26.*t74.*t177.*5.184613271881752e-2+t2.*t26.*t75.*t177.*2.592306635940876e-2-t26.*t27.*t74.*t177.*5.184613271881752e-2-t26.*t44.*t74.*t177.*5.184613271881752e-2+t26.*t44.*t75.*t177.*2.592306635940876e-2+t2.*t26.*t176.*t177.*5.184613271881752e-2-t2.*t26.*t177.*t179.*1.555383981564525e-1+t26.*t44.*t176.*t177.*5.184613271881752e-2+t2.*t74.*t174.*t175.*5.184613271881752e-2-t2.*t75.*t174.*t175.*2.592306635940876e-2-t26.*t44.*t177.*t179.*1.555383981564525e-1-t2.*t75.*t178.*t184.*1.03692265437635e-1+t27.*t74.*t174.*t175.*5.184613271881752e-2+t44.*t74.*t174.*t175.*5.184613271881752e-2-t44.*t75.*t174.*t175.*2.592306635940876e-2-t44.*t75.*t178.*t184.*1.03692265437635e-1-t2.*t174.*t175.*t176.*5.184613271881752e-2+t2.*t174.*t175.*t179.*1.555383981564525e-1-t2.*t176.*t178.*t184.*5.184613271881752e-2-t2.*t178.*t179.*t184.*5.184613271881752e-2-t44.*t174.*t175.*t176.*5.184613271881752e-2+t44.*t174.*t175.*t179.*1.555383981564525e-1-t44.*t176.*t178.*t184.*5.184613271881752e-2-t44.*t178.*t179.*t184.*5.184613271881752e-2+deltap_i.*phip_i.*t26.*t175.*t185.*1.03692265437635e-1+deltap_i.*phip_i.*t174.*t177.*t185.*1.03692265437635e-1-deltap_i.*t26.*t74.*t177.*thetap.*1.03692265437635e-1+deltap_i.*t26.*t75.*t177.*thetap.*5.184613271881752e-2+deltap_i.*t26.*t176.*t177.*thetap.*1.03692265437635e-1-deltap_i.*t26.*t177.*t179.*thetap.*3.110767963129051e-1+deltap_i.*t74.*t174.*t175.*thetap.*1.03692265437635e-1-deltap_i.*t75.*t174.*t175.*thetap.*5.184613271881752e-2-deltap_i.*t75.*t178.*t184.*thetap.*2.073845308752701e-1-deltap_i.*t174.*t175.*t176.*thetap.*1.03692265437635e-1+deltap_i.*t174.*t175.*t179.*thetap.*3.110767963129051e-1-deltap_i.*t176.*t178.*t184.*thetap.*1.03692265437635e-1-deltap_i.*t178.*t179.*t184.*thetap.*1.03692265437635e-1+phip_i.*t26.*t175.*t185.*thetap.*1.03692265437635e-1+phip_i.*t174.*t177.*t185.*thetap.*1.03692265437635e-1+t2.*t3.*t4.*t7.*t75.*t184.*4.666151944693576e-1+t3.*t4.*t7.*t44.*t75.*t184.*4.666151944693576e-1+t2.*t3.*t4.*t7.*t176.*t184.*2.333075972346788e-1+t2.*t3.*t4.*t7.*t179.*t184.*2.333075972346788e-1+t3.*t4.*t7.*t44.*t176.*t184.*2.333075972346788e-1+t3.*t4.*t7.*t44.*t179.*t184.*2.333075972346788e-1+deltap_i.*t3.*t4.*t7.*t75.*t184.*thetap.*9.332303889387153e-1+deltap_i.*t3.*t4.*t7.*t176.*t184.*thetap.*4.666151944693576e-1+deltap_i.*t3.*t4.*t7.*t179.*t184.*thetap.*4.666151944693576e-1;f_phi_o-t2.*t76.*5.184613271881752e-2-t2.*t77.*7.776919907822627e-2-t15.*t76.*5.184613271881752e-2-t17.*t76.*5.184613271881752e-2-t17.*t77.*7.776919907822627e-2-deltap_o.*t76.*thetap.*1.03692265437635e-1-deltap_o.*t77.*thetap.*1.555383981564525e-1-deltap_o.*phip_o.*t26.*t189.*1.03692265437635e-1-deltap_o.*phip_o.*t174.*t191.*1.03692265437635e-1-phip_o.*t26.*t189.*thetap.*1.03692265437635e-1-phip_o.*t174.*t191.*thetap.*1.03692265437635e-1+t2.*t3.*t77.*t188.*1.03692265437635e-1+t3.*t17.*t77.*t188.*1.03692265437635e-1-t2.*t26.*t76.*t191.*5.184613271881752e-2+t2.*t26.*t77.*t191.*2.592306635940876e-2-t15.*t26.*t76.*t191.*5.184613271881752e-2-t17.*t26.*t76.*t191.*5.184613271881752e-2+t17.*t26.*t77.*t191.*2.592306635940876e-2+t2.*t3.*t187.*t188.*5.184613271881752e-2+t2.*t3.*t188.*t190.*5.184613271881752e-2+t3.*t17.*t187.*t188.*5.184613271881752e-2+t3.*t17.*t188.*t190.*5.184613271881752e-2+t2.*t26.*t187.*t191.*5.184613271881752e-2-t2.*t26.*t190.*t191.*1.555383981564525e-1+t17.*t26.*t187.*t191.*5.184613271881752e-2-t17.*t26.*t190.*t191.*1.555383981564525e-1+t2.*t76.*t174.*t189.*5.184613271881752e-2-t2.*t77.*t174.*t189.*2.592306635940876e-2-t2.*t77.*t178.*t186.*1.03692265437635e-1+t15.*t76.*t174.*t189.*5.184613271881752e-2+t17.*t76.*t174.*t189.*5.184613271881752e-2-t17.*t77.*t174.*t189.*2.592306635940876e-2-t17.*t77.*t178.*t186.*1.03692265437635e-1-t2.*t174.*t187.*t189.*5.184613271881752e-2-t2.*t178.*t186.*t187.*5.184613271881752e-2+t2.*t174.*t189.*t190.*1.555383981564525e-1-t2.*t178.*t186.*t190.*5.184613271881752e-2-t17.*t174.*t187.*t189.*5.184613271881752e-2-t17.*t178.*t186.*t187.*5.184613271881752e-2+t17.*t174.*t189.*t190.*1.555383981564525e-1-t17.*t178.*t186.*t190.*5.184613271881752e-2+deltap_o.*phip_o.*t26.*t189.*t192.*1.03692265437635e-1+deltap_o.*phip_o.*t174.*t191.*t192.*1.03692265437635e-1+deltap_o.*t3.*t77.*t188.*thetap.*2.073845308752701e-1-deltap_o.*t26.*t76.*t191.*thetap.*1.03692265437635e-1+deltap_o.*t26.*t77.*t191.*thetap.*5.184613271881752e-2+deltap_o.*t3.*t187.*t188.*thetap.*1.03692265437635e-1+deltap_o.*t3.*t188.*t190.*thetap.*1.03692265437635e-1+deltap_o.*t26.*t187.*t191.*thetap.*1.03692265437635e-1-deltap_o.*t26.*t190.*t191.*thetap.*3.110767963129051e-1+deltap_o.*t76.*t174.*t189.*thetap.*1.03692265437635e-1-deltap_o.*t77.*t174.*t189.*thetap.*5.184613271881752e-2-deltap_o.*t77.*t178.*t186.*thetap.*2.073845308752701e-1-deltap_o.*t174.*t187.*t189.*thetap.*1.03692265437635e-1-deltap_o.*t178.*t186.*t187.*thetap.*1.03692265437635e-1+deltap_o.*t174.*t189.*t190.*thetap.*3.110767963129051e-1-deltap_o.*t178.*t186.*t190.*thetap.*1.03692265437635e-1+phip_o.*t26.*t189.*t192.*thetap.*1.03692265437635e-1+phip_o.*t174.*t191.*t192.*thetap.*1.03692265437635e-1;f_phi_r-t2.*t193.*t197.*2.073845308752701e-1+t2.*t193.*t198.*2.073845308752701e-1+phip_r.*t3.*t178.*thetap.*4.147690617505401e-1-t2.*t178.*t193.*t196.*2.073845308752701e-1-t2.*t193.*t194.*t195.*2.073845308752701e-1+t2.*t193.*t194.*t197.*4.147690617505401e-1-t2.*t193.*t195.*t196.*6.221535926258102e-1-t2.*t193.*t194.*t198.*4.147690617505401e-1+t2.*t193.*t195.*t198.*2.073845308752701e-1+t2.*t193.*t196.*t197.*2.073845308752701e-1-t2.*t193.*t196.*t198.*2.073845308752701e-1-t14.*t193.*t195.*t198.*2.073845308752701e-1-phip_r.*t3.*t178.*t194.*thetap.*8.295381235010802e-1-phip_r.*t3.*t178.*t196.*thetap.*4.147690617505401e-1+t2.*t178.*t193.*t194.*t195.*4.147690617505401e-1-t2.*t178.*t193.*t195.*t196.*4.147690617505401e-1+t2.*t193.*t194.*t195.*t197.*6.221535926258102e-1+t2.*t193.*t195.*t196.*t197.*2.073845308752701e-1;f_phi_l-t2.*t197.*t199.*2.073845308752701e-1+t2.*t198.*t199.*2.073845308752701e-1+phip_l.*t3.*t178.*thetap.*4.147690617505401e-1-t2.*t178.*t199.*t202.*2.073845308752701e-1+t2.*t197.*t199.*t200.*4.147690617505401e-1-t2.*t198.*t199.*t200.*4.147690617505401e-1+t2.*t197.*t199.*t202.*2.073845308752701e-1+t2.*t198.*t199.*t201.*2.073845308752701e-1-t2.*t198.*t199.*t202.*2.073845308752701e-1-t2.*t199.*t200.*t201.*2.073845308752701e-1-t2.*t199.*t201.*t202.*6.221535926258102e-1-t12.*t198.*t199.*t201.*2.073845308752701e-1-phip_l.*t3.*t178.*t200.*thetap.*8.295381235010802e-1-phip_l.*t3.*t178.*t202.*thetap.*4.147690617505401e-1+t2.*t178.*t199.*t200.*t201.*4.147690617505401e-1-t2.*t178.*t199.*t201.*t202.*4.147690617505401e-1+t2.*t197.*t199.*t200.*t201.*6.221535926258102e-1+t2.*t197.*t199.*t201.*t202.*2.073845308752701e-1];

end

== matlab function car_model/Vehicle/Steering_model/Auxiliary_matrices/dA_matrix ==
  data: in1 input; dA output
function dA = dConstraintMatrix(in1)

%    This function was generated by the Symbolic Math Toolbox version 7.2.

%    11-Nov-2020 11:00:02



delta_o = in1(5,:);

p1 = in1(10,:);

p2 = in1(11,:);

theta = in1(3,:);

t2 = tan(theta);

t3 = t2.^2;

t4 = t2.*(3.0./2.0);

t5 = t4+9.0./2.0;

t6 = t3+1.0;

t7 = 1.0./t5.^2;

t8 = tan(delta_o);

t9 = t8.^2;

t10 = t9+1.0;

t11 = 1.0./t5;

t12 = t3.*t7.*(8.1e1./4.0);

t13 = t12+1.0;

t14 = 1.0./t5.^3;

t15 = t2.*t6.*t7.*(8.1e1./2.0);

t16 = t6.*t11.*(2.7e1./4.0);

t21 = t2.*t6.*t7.*(8.1e1./8.0);

t17 = t16-t21;

t18 = t2.*t11.*(2.7e1./4.0);

t19 = cos(delta_o);

t20 = 1.0./t19;

t22 = t18+9.0;

t23 = t18-9.0;

t24 = 1.0./t22;

t25 = t2.*t11.*(9.0./2.0);

t26 = atan(t25);

t27 = t26+theta;

t28 = 1.0./t13;

t29 = t6.*t11.*(9.0./2.0);

t38 = t2.*t6.*t7.*(2.7e1./4.0);

t30 = t29-t38;

t31 = t28.*t30;

t32 = t31+1.0;

t36 = t3.*t6.*t14.*(2.43e2./4.0);

t33 = t15-t36;

t34 = 1.0./sqrt(t13);

t35 = 1.0./t13.^(3.0./2.0);

t37 = cos(t27);

t39 = p1.*t32.*t37;

t40 = sin(t27);

dA = reshape([0.0,0.0,0.0,-p1.*t32.*t40,-t39,0.0,0.0,0.0,t39,-p1.*t32.*t40,0.0,0.0,0.0,p1.*(t33.*t35.*(9.0./4.0)+t6.*t11.*t34.*(2.7e1./8.0)-t2.*t6.*t7.*t34.*(8.1e1./1.6e1)-t2.*t11.*t35.*(t15-t36).*(2.7e1./1.6e1)),-p1.*(t33.*t35.*(3.0./8.0)-t6.*t11.*t34.*(8.1e1./4.0)+t2.*t6.*t7.*t34.*(2.43e2./8.0)+t2.*t11.*t33.*t35.*(8.1e1./8.0)),p1.*t33.*(t8.*(3.0./2.0)-9.0./2.0).*(-2.0./9.0)-p2.*t10.*t13.*(1.0./3.0),0.0,0.0,0.0,0.0,p1.*t10.*t17.*(-2.0./9.0)-p2.*t8.*t10.*(t18+9.0./2.0).*(4.0./9.0),0.0,0.0,0.0,0.0,0.0,0.0,p1.*t33.*t34.*(1.0./2.0),0.0,0.0,0.0,0.0,p1.*(t17.*t20.*t24-t17.*t20.*1.0./t22.^2.*t23)+p2.*1.0./t19.^2.*t23.*t24.*sin(delta_o),0.0,0.0,0.0,-p1.*(t6.*t11.*(3.0./2.0)-t2.*t6.*t7.*(9.0./4.0)),0.0,0.0,0.0,0.0,0.0,0.0,0.0,0.0],[5,9]);

end
